simulink model "final_quadruped_140622_veldelay"  (R2021a)
settings: Solver=ode15s  StartTime=0.0  StopTime=10  FixedStep=1e-3  RelTol=1e-5  EnableMultiTasking=on
values from neighbouring files (symbols this model uses):
  foot_x = 8    [bipedparameters.m]    (also in fcn.m; finalrobotParameters.m; finalrobotParameters_110522.m; finalrobotParameters_140522.m)
  foot_y = 6    [bipedparameters.m]    (also in fcn.m; finalrobotParameters.m; finalrobotParameters_110522.m; finalrobotParameters_140522.m)
  foot_z = 1    [bipedparameters.m]    (also in fcn.m; finalrobotParameters.m; finalrobotParameters_110522.m; finalrobotParameters_140522.m)
  height_plane = 0.025    [bipedparameters.m]    (also in finalrobotParameters.m; finalrobotParameters_110522.m; finalrobotParameters_140522.m; finalrobotParameters_240522.m)
  kd_ankle = 1000    [bipedparameters.m]    (also in finalrobotParameters_240522.m)
  kd_hip = 1000    [bipedparameters.m]    (also in finalrobotParameters_240522.m)
  kd_knee = 1000    [bipedparameters.m]    (also in finalrobotParameters_240522.m)
  ki_ankle = 1000    [bipedparameters.m]    (also in finalrobotParameters_240522.m)
  ki_hip = 1000    [bipedparameters.m]    (also in finalrobotParameters_240522.m)
  ki_knee = 2000    [bipedparameters.m]    (also in finalrobotParameters_240522.m)
  kp_ankle = 1000    [bipedparameters.m]    (also in finalrobotParameters_240522.m)
  kp_hip = 1000    [bipedparameters.m]    (also in finalrobotParameters_240522.m)
  kp_knee = 2000    [bipedparameters.m]    (also in finalrobotParameters_240522.m)
  lower_leg_length = 10    [bipedparameters.m]    (also in fcn.m; finalrobotParameters.m; finalrobotParameters_110522.m; finalrobotParameters_140522.m)
  m_ll = density*leg_radius*leg_radius*lower_leg_length*3.141592653589*0.01*0.01*0.01    (= 0.0176714586764)    [bipedparameters.m]    (also in fcn.m; finalrobotParameters_140522.m; finalrobotParameters_240522.m; hdotlb.m)
  m_ul = density*leg_radius*leg_radius*upper_leg_length*3.141592653589*0.01*0.01*0.01    (= 0.0176714586764)    [bipedparameters.m]    (also in fcn.m; finalrobotParameters_140522.m; finalrobotParameters_240522.m; hdotlb.m)
  plane_x = 25    [bipedparameters.m]    (also in finalrobotParameters.m; finalrobotParameters_110522.m; finalrobotParameters_140522.m; finalrobotParameters_240522.m)
  plane_y = 3    [bipedparameters.m]    (also in finalrobotParameters.m; finalrobotParameters_110522.m; finalrobotParameters_140522.m; finalrobotParameters_240522.m)
  torso_offset_x = -0.5    [bipedparameters.m]    (also in finalrobotParameters.m = 10; finalrobotParameters_110522.m = 10; finalrobotParameters_140522.m = 10; finalrobotParameters_240522.m = 10)
  torso_offset_z = -2    [bipedparameters.m]    (also in finalrobotParameters.m; finalrobotParameters_110522.m; finalrobotParameters_140522.m; finalrobotParameters_240522.m)
  torso_x = 5    [bipedparameters.m]    (also in fcn.m = 25; finalrobotParameters.m = 25; finalrobotParameters_110522.m = 25; finalrobotParameters_140522.m = 25)
  torso_y = 10    [bipedparameters.m]    (also in fcn.m = 16; finalrobotParameters.m = 16; finalrobotParameters_110522.m = 16; finalrobotParameters_140522.m = 16)
  torso_z = 8    [bipedparameters.m]    (also in fcn.m = 10; finalrobotParameters.m = 10; finalrobotParameters_110522.m = 10; finalrobotParameters_140522.m = 10)
  upper_leg_length = 10    [bipedparameters.m]    (also in fcn.m; finalrobotParameters.m; finalrobotParameters_110522.m; finalrobotParameters_140522.m)
undefined symbols (not defined in the file or in its folder): X, Y, Z
libraries: nesl_utility x151, sm_lib x71, Contact_Forces_Lib x16, pid_lib x12, fl_lib x4
(part 7 of 7)

== matlab function final_quadruped_140622_veldelay/Model/Left Leg Front/Subsystem/MATLAB Function1 ==
  data: eb10g input; eb20g input; ab10g input; cmb2 input; cmb1 input; cmb3 input; eb30g input; hLF output; ab20g input; rhoLF output
function [hLF,rhoLF] = fcn(eb10g, eb20g, ab10g, cmb2, cmb1, cmb3, eb30g, ab20g)
%%
lower_leg_length = 10;
upper_leg_length = 10;
density = 1000;
foot_density=2000;
leg_radius = 0.75;
foot_x = 8;
foot_y = 6;
foot_z = 1;
m_ul=density*leg_radius*leg_radius*upper_leg_length*3.141592653589*0.01*0.01*0.01;
m_ll=density*leg_radius*leg_radius*lower_leg_length*3.141592653589*0.01*0.01*0.01;
m_foot=foot_density*foot_x*foot_y*foot_z*0.000001;
%%
scf=zeros(3,3);
sof=zeros(3,3);
rhoLF=zeros(3,3,3);
scf(:,1)=cmb1;
scf(:,2)=ab10g+cmb2;
scf(:,3)=ab10g+ab20g+cmb3;
sof(:,1)=[0;0;0];
sof(:,2)=ab10g;
sof(:,3)=ab10g+ab20g;
for i=1:3
    for j=1:3
        if j<i
rhoLF(:,j,i)=zeros(3,1);
        else
rhoLF(:,j,i)=scf(:,j)-sof(:,i);
        end
    end
end
h1=(m_ul*cross(eb10g,rhoLF(:,1,1)))+(m_ll*cross(eb10g,rhoLF(:,2,1)))+(m_foot*cross(eb10g,rhoLF(:,3,1)));
h2=(m_ll*cross(eb20g,rhoLF(:,2,2)))+(m_foot*cross(eb20g,rhoLF(:,3,2)));
h3=m_foot*(cross(eb30g,rhoLF(:,3,3)));

hLF =[h1 h2 h3];



end

== matlab function final_quadruped_140622_veldelay/Model/Right Leg Back/Subsystem/MATLAB Function1 ==
  data: ec10g input; ec20g input; ac10g input; cmc2 input; cmc1 input; cmc3 input; ec30g input; ac20g input; hRB output; rhoRB output
function [hRB,rhoRB] = fcn(ec10g, ec20g, ac10g, cmc2, cmc1, cmc3, ec30g, ac20g)
%%
lower_leg_length = 10;
upper_leg_length = 10;
density = 1000;
foot_density=2000;
leg_radius = 0.75;
foot_x = 8;
foot_y = 6;
foot_z = 1;
m_ul=density*leg_radius*leg_radius*upper_leg_length*3.141592653589*0.01*0.01*0.01;
m_ll=density*leg_radius*leg_radius*lower_leg_length*3.141592653589*0.01*0.01*0.01;
m_foot=foot_density*foot_x*foot_y*foot_z*0.000001;
%%
scf=zeros(3,3);
sof=zeros(3,3);
rhoRB=zeros(3,3,3);
scf(:,1)=cmc1;
scf(:,2)=ac10g+cmc2;
scf(:,3)=ac10g+ac20g+cmc3;
sof(:,1)=[0;0;0];
sof(:,2)=ac10g;
sof(:,3)=ac10g+ac20g;
for i=1:3
    for j=1:3
        if j<i
rhoRB(:,j,i)=zeros(3,1);
        else
rhoRB(:,j,i)=scf(:,j)-sof(:,i);
        end
    end
end
h1=(m_ul*cross(ec10g,rhoRB(:,1,1)))+(m_ll*cross(ec10g,rhoRB(:,2,1)))+(m_foot*cross(ec10g,rhoRB(:,3,1)));
h2=(m_ll*cross(ec20g,rhoRB(:,2,2)))+(m_foot*cross(ec20g,rhoRB(:,3,2)));
h3=m_foot*(cross(ec30g,rhoRB(:,3,3)));

hRB =[h1 h2 h3];



end

== matlab function final_quadruped_140622_veldelay/Model/Left LegBack/Subsystem/MATLAB Function1 ==
  data: ed10g input; ed20g input; ad10g input; cmd2 input; cmd1 input; cmd3 input; ed30g input; ad20g input; hLB output; rhoLB output
function [hLB,rhoLB] = fcn(ed10g, ed20g, ad10g, cmd2, cmd1, cmd3, ed30g, ad20g)
%%
lower_leg_length = 10;
upper_leg_length = 10;
density = 1000;
foot_density=2000;
leg_radius = 0.75;
foot_x = 8;
foot_y = 6;
foot_z = 1;
m_ul=density*leg_radius*leg_radius*upper_leg_length*3.141592653589*0.01*0.01*0.01;
m_ll=density*leg_radius*leg_radius*lower_leg_length*3.141592653589*0.01*0.01*0.01;
m_foot=foot_density*foot_x*foot_y*foot_z*0.000001;
%%
scf=zeros(3,3);
sof=zeros(3,3);
rhoLB=zeros(3,3,3);
scf(:,1)=cmd1;
scf(:,2)=ad10g+cmd2;
scf(:,3)=ad10g+ad20g+cmd3;
sof(:,1)=[0;0;0];
sof(:,2)=ad10g;
sof(:,3)=ad10g+ad20g;
for i=1:3
    for j=1:3
        if j<i
rhoLB(:,j,i)=zeros(3,1);
        else
rhoLB(:,j,i)=scf(:,j)-sof(:,i);
        end
    end
end
h1=(m_ul*cross(ed10g,rhoLB(:,1,1)))+(m_ll*cross(ed10g,rhoLB(:,2,1)))+(m_foot*cross(ed10g,rhoLB(:,3,1)));
h2=(m_ll*cross(ed20g,rhoLB(:,2,2)))+(m_foot*cross(ed20g,rhoLB(:,3,2)));
h3=m_foot*(cross(ed30g,rhoLB(:,3,3)));

hLB =[h1 h2 h3];



end

== matlab function final_quadruped_140622_veldelay/MATLAB Function ==
  data: vx input; v_torso output; vy input; vz input
function v_torso = fcn(vx, vy, vz)
v_torso=[vx; vy; vz];
end

== matlab function final_quadruped_140622_veldelay/Model/Right Leg Front /MATLAB Function2 ==
  data: tddRF input; tddRF_hip output; tddRF_knee output; tddRF_ankle output
function [tddRF_hip, tddRF_knee, tddRF_ankle] = fcn(tddRF)
tddRF_hip=tddRF(1);
tddRF_knee=tddRF(2);
tddRF_ankle=tddRF(3);
end

== matlab function final_quadruped_140622_veldelay/Model/Left Leg Front/MATLAB Function2 ==
  data: tddLF input; tddLF_hip output; tddLF_knee output; tddLF_ankle output
function [tddLF_hip, tddLF_knee, tddLF_ankle] = fcn(tddLF)
tddLF_hip=tddLF(1);
tddLF_knee=tddLF(2);
tddLF_ankle=tddLF(3);
end

== matlab function final_quadruped_140622_veldelay/Model/Right Leg Back/MATLAB Function2 ==
  data: tddRB input; tddRB_hip output; tddRB_knee output; tddRB_ankle output
function [tddRB_hip, tddRB_knee, tddRB_ankle] = fcn(tddRB)
tddRB_hip=tddRB(1);
tddRB_knee=tddRB(2);
tddRB_ankle=tddRB(3);
end

== matlab function final_quadruped_140622_veldelay/Model/Left LegBack/MATLAB Function2 ==
  data: tddLB input; tddLB_hip output; tddLB_knee output; tddLB_ankle output
function [tddLB_hip, tddLB_knee, tddLB_ankle] = fcn(tddLB)
tddLB_hip=tddLB(1);
tddLB_knee=tddLB(2);
tddLB_ankle=tddLB(3);
end

== matlab function final_quadruped_140622_veldelay/Subsystem/MATLAB Function4 ==
  data: vx input; vy input; v output; vz input; ax input; ay input; az input; a output
function [v,a] = fcn(vx,vy,vz,ax,ay,az)
v=[vx;vy;vz];
a=[ax;ay;az];
end

== matlab function final_quadruped_140622_veldelay/Subsystem/MATLAB Function1 ==
  data: vx input; vy input; v output; vz input; ax input; ay input; az input; a output
function [v,a] = fcn(vx,vy,vz,ax,ay,az)
v=[vx;vy;vz];
a=[ax;ay;az];
end

== matlab function final_quadruped_140622_veldelay/Subsystem/MATLAB Function5 ==
  data: vx input; vy input; v output; vz input; ax input; ay input; az input; a output
function [v,a] = fcn(vx,vy,vz,ax,ay,az)
v=[vx;vy;vz];
a=[ax;ay;az];
end

== matlab function final_quadruped_140622_veldelay/Subsystem/MATLAB Function6 ==
  data: vx input; vy input; v output; vz input; ax input; ay input; az input; a output
function [v,a] = fcn(vx,vy,vz,ax,ay,az)
v=[vx;vy;vz];
a=[ax;ay;az];
end

== matlab function final_quadruped_140622_veldelay/Subsystem/MATLAB Function7 ==
  data: vx input; vy input; v output; vz input; ax input; ay input; az input; a output
function [v,a] = fcn(vx,vy,vz,ax,ay,az)
v=[vx;vy;vz];
a=[ax;ay;az];
end

== matlab function final_quadruped_140622_veldelay/Subsystem/MATLAB Function8 ==
  data: vx input; vy input; v output; vz input; ax input; ay input; az input; a output
function [v,a] = fcn(vx,vy,vz,ax,ay,az)
v=[vx;vy;vz];
a=[ax;ay;az];
end

== matlab function final_quadruped_140622_veldelay/Subsystem/MATLAB Function9 ==
  data: vx input; vy input; v output; vz input; ax input; ay input; az input; a output
function [v,a] = fcn(vx,vy,vz,ax,ay,az)
v=[vx;vy;vz];
a=[ax;ay;az];
end

== matlab function final_quadruped_140622_veldelay/Subsystem/MATLAB Function10 ==
  data: vx input; vy input; v output; vz input; ax input; ay input; az input; a output
function [v,a] = fcn(vx,vy,vz,ax,ay,az)
v=[vx;vy;vz];
a=[ax;ay;az];
end

== matlab function final_quadruped_140622_veldelay/Subsystem/MATLAB Function11 ==
  data: vx input; vy input; v output; vz input; ax input; ay input; az input; a output
function [v,a] = fcn(vx,vy,vz,ax,ay,az)
v=[vx;vy;vz];
a=[ax;ay;az];
end

== matlab function final_quadruped_140622_veldelay/Subsystem/MATLAB Function12 ==
  data: vx input; vy input; v output; vz input; ax input; ay input; az input; a output
function [v,a] = fcn(vx,vy,vz,ax,ay,az)
v=[vx;vy;vz];
a=[ax;ay;az];
end

== matlab function final_quadruped_140622_veldelay/Subsystem/MATLAB Function14 ==
  data: vx input; vy input; v output; vz input; ax input; ay input; az input; a output
function [v,a] = fcn(vx,vy,vz,ax,ay,az)
v=[vx;vy;vz];
a=[ax;ay;az];
end

== matlab function final_quadruped_140622_veldelay/Model/Right Leg Front /MATLAB Function ==
  data: ankle input; knee input; tdRF output; hip input
function tdRF= fcn(ankle, knee, hip)
tdRF=[hip;knee;ankle];
end

== matlab function final_quadruped_140622_veldelay/Subsystem/MATLAB Function13 ==
  data: vulRF input; vllRF input; Mvcm output; vfRF input; vulLF input; vllLF input; vfLF input; vulRB input; vllRB input; vfRB input; vulLB input; vllLB input; vfLB input; v_torso input; vlinks output; vcm output
function [Mvcm,vlinks,vcm] = fcn(vulRF,vllRF,vfRF,vulLF,vllLF,vfLF,vulRB,vllRB,vfRB,vulLB,vllLB,vfLB,v_torso)
%%
lower_leg_length = 10;
upper_leg_length = 10;
density = 1000;
foot_density=2000;
leg_radius = 0.75;
foot_x = 8;
foot_y = 6;
foot_z = 1;
torso_y = 16;
torso_x = 25;
torso_z = 10;
m_ul=density*leg_radius*leg_radius*upper_leg_length*3.141592653589*0.01*0.01*0.01;
m_ll=density*leg_radius*leg_radius*lower_leg_length*3.141592653589*0.01*0.01*0.01;
m_foot=foot_density*foot_x*foot_y*foot_z*0.000001;
m_torso=density*torso_x*torso_y*torso_z*0.000001;
M=m_torso+4*(m_ul+m_ll+m_foot);
%%
Mvcm=m_torso*v_torso+(m_ul*vulRF+m_ll*vllRF+m_foot*vfRF)+(m_ul*vulLF+m_ll*vllLF+m_foot*vfLF)+(m_ul*vulRB+m_ll*vllRB+m_foot*vfRB)+(m_ul*vulLB+m_ll*vllLB+m_foot*vfLB);
vlinks=[vulRF vllRF vfRF vulLF vllLF vfLF vulRB vllRB vfRB vulLB vllLB vfLB];
vcm=Mvcm/M;
end

== matlab function final_quadruped_140622_veldelay/Model/Left Leg Front/MATLAB Function ==
  data: ankle input; knee input; tdRF output; hip input
function tdRF= fcn(ankle, knee, hip)
tdRF=[hip;knee;ankle];
end

== matlab function final_quadruped_140622_veldelay/Model/Right Leg Back/MATLAB Function ==
  data: ankle input; knee input; tdRF output; hip input
function tdRF= fcn(ankle, knee, hip)
tdRF=[hip;knee;ankle];
end

== matlab function final_quadruped_140622_veldelay/Model/Left LegBack/MATLAB Function ==
  data: ankle input; knee input; tdLB output; hip input
function tdLB= fcn(ankle, knee, hip)
tdLB=[hip;knee;ankle];
end

== matlab function final_quadruped_140622_veldelay/Model/MATLAB Function ==
  data: tdRF input; td output; tdLF input; tdRB input; tdLB input; t2dRF input; t2dLF input; t2dRB input; t2dLB input; t2d output
function [td,t2d] = fcn(tdRF,tdLF,tdRB,tdLB,t2dRF,t2dLF,t2dRB,t2dLB)
td=[tdRF;tdLF;tdRB;tdLB];
t2d=[t2dRF;t2dLF;t2dRB;t2dLB];
end

== matlab function final_quadruped_140622_veldelay/Model/MATLAB Function1 ==
  data: h input; h_dot input; ht2d output; td input; t2d input; h_dottd output; htd output; theta_d_des input; theta_2d_des input; ht2ddes output; hdtddes output
function [ht2d,h_dottd,htd,ht2ddes,hdtddes] = fcn(h,h_dot, td, t2d,theta_d_des,theta_2d_des)
ht2d=h*t2d;
htd=h*td;
h_dottd=h_dot*td;
ht2ddes=h*theta_2d_des;
hdtddes=h_dot*theta_d_des;
end

== matlab function final_quadruped_140622_veldelay/MATLAB Function1 ==
  data: Mvcm input; error output; ht2d input; h_dottd input; a_torso input; v_torso input; f input; Macm input; htd input; ht2ddes input; hdtddes input; v_error output; theta_d_des input; h input; v_error_eig output
function [error, v_error,v_error_eig] = fcn(Mvcm,ht2d,h_dottd,a_torso, v_torso, f,Macm,htd, ht2ddes, hdtddes, theta_d_des,h)
%%
lower_leg_length = 10;
upper_leg_length = 10;
density = 1000;
foot_density=2000;
leg_radius = 0.75;
foot_x = 8;
foot_y = 6;
foot_z = 1;
torso_y = 16;
torso_x = 25;
torso_z = 10;
m_ul=density*leg_radius*leg_radius*upper_leg_length*3.141592653589*0.01*0.01*0.01;
m_ll=density*leg_radius*leg_radius*lower_leg_length*3.141592653589*0.01*0.01*0.01;
m_foot=foot_density*foot_x*foot_y*foot_z*0.000001;
m_torso=density*torso_x*torso_y*torso_z*0.000001;
M=m_torso+(4*(m_ul+m_ll+m_foot));
g=[0; 0; -9.80067];
%%
%v_error=htd+M*v_torso-Mvcm;
v_error=h*theta_d_des+M*v_torso-Mvcm;
v_error_eig=h*theta_d_des+M*v_torso-Mvcm;
error2=ht2d+h_dottd+M*a_torso-M*g-f-Macm;
error=ht2ddes+hdtddes+M*a_torso-M*g-f-Macm;
end

== matlab function final_quadruped_140622_veldelay/Model/Right Leg Front /Subsystem/MATLAB Function2 ==
  data: h_dotRF output; ea_dg1 input; ea1g input; ea2g input; ea3g input; ea_dg2 input; ea_dg3 input; rho_dotRF input; rhoRF input
function h_dotRF = fcn(  ea_dg1,ea1g, ea2g, ea3g, ea_dg2, ea_dg3, rho_dotRF, rhoRF)
%%
lower_leg_length = 10;
upper_leg_length = 10;
density = 1000;
foot_density=2000;
leg_radius = 0.75;
foot_x = 8;
foot_y = 6;
foot_z = 1;
m_ul=density*leg_radius*leg_radius*upper_leg_length*3.141592653589*0.01*0.01*0.01;
m_ll=density*leg_radius*leg_radius*lower_leg_length*3.141592653589*0.01*0.01*0.01;
m_foot=foot_density*foot_x*foot_y*foot_z*0.000001;

%%
h1_dot=(m_ul*cross(ea1g,rho_dotRF(:,1,1)))+(m_ul*cross(ea_dg1,rhoRF(:,1,1)))+(m_ll*cross(ea1g,rho_dotRF(:,2,1)))+(m_ll*cross(ea_dg1,rhoRF(:,2,1)))+(m_foot*cross(ea1g,rho_dotRF(:,3,1)))+(m_foot*cross(ea_dg1,rhoRF(:,3,1)));
h2_dot=(m_ll*cross(ea2g,rho_dotRF(:,2,2)))+(m_ll*cross(ea_dg2,rhoRF(:,2,2)))+(m_foot*cross(ea2g,rho_dotRF(:,3,2)))+(m_foot*cross(ea_dg2,rhoRF(:,3,2)));
h3_dot=m_foot*(cross(ea3g,rho_dotRF(:,3,3)))+m_foot*(cross(ea_dg3,rhoRF(:,3,3)));

h_dotRF =[h1_dot h2_dot h3_dot];



end

== matlab function final_quadruped_140622_veldelay/Model/Left Leg Front/Subsystem/MATLAB Function2 ==
  data: h_dotLF output; eb_dg1 input; eb1g input; eb2g input; eb3g input; eb_dg2 input; eb_dg3 input; rho_dotLF input; rhoLF input
function h_dotLF = fcn( eb_dg1,eb1g, eb2g, eb3g, eb_dg2, eb_dg3, rho_dotLF, rhoLF)
%%
lower_leg_length = 10;
upper_leg_length = 10;
density = 1000;
foot_density=2000;
leg_radius = 0.75;
foot_x = 8;
foot_y = 6;
foot_z = 1;
m_ul=density*leg_radius*leg_radius*upper_leg_length*3.141592653589*0.01*0.01*0.01;
m_ll=density*leg_radius*leg_radius*lower_leg_length*3.141592653589*0.01*0.01*0.01;
m_foot=foot_density*foot_x*foot_y*foot_z*0.000001;

%%
h1_dot=(m_ul*cross(eb1g,rho_dotLF(:,1,1)))+(m_ul*cross(eb_dg1,rhoLF(:,1,1)))+(m_ll*cross(eb1g,rho_dotLF(:,2,1)))+(m_ll*cross(eb_dg1,rhoLF(:,2,1)))+(m_foot*cross(eb1g,rho_dotLF(:,3,1)))+(m_foot*cross(eb_dg1,rhoLF(:,3,1)));
h2_dot=(m_ll*cross(eb2g,rho_dotLF(:,2,2)))+(m_ll*cross(eb_dg2,rhoLF(:,2,2)))+(m_foot*cross(eb2g,rho_dotLF(:,3,2)))+(m_foot*cross(eb_dg2,rhoLF(:,3,2)));
h3_dot=m_foot*(cross(eb3g,rho_dotLF(:,3,3)))+m_foot*(cross(eb_dg3,rhoLF(:,3,3)));

h_dotLF =[h1_dot h2_dot h3_dot];



end

== matlab function final_quadruped_140622_veldelay/Model/Right Leg Front /Subsystem/MATLAB Function4 ==
  data: ea1g input; ea2g input; aa1g input; aa2g input; ea3g input; vlinks input; w_torso input; ea_dg1 output; td1 input; v_torso input; ea_dg2 output; td2 input; td3 input; ea_dg3 output; rho_dotRF output
function [ea_dg1,ea_dg2,ea_dg3,rho_dotRF] = fcn(ea1g,ea2g,aa1g,aa2g, ea3g, vlinks, w_torso, td1, v_torso, td2, td3)
w0=w_torso;
w1=w0+ea1g*td1;
w2=w1+ea2g*td2;
w3=w2+ea3g*td3;
%e dot = omega X e
ea_dg1=cross(w1,ea1g);
ea_dg2=cross(w2,ea2g);
ea_dg3=cross(w3,ea3g);


vcf=zeros(3,3);
vof=zeros(3,3);
rho_dotRF=zeros(3,3,3);
vcf(:,1)=vlinks(1);
vcf(:,2)=vlinks(2);
vcf(:,3)=vlinks(3);
vof(:,1)=v_torso;
vof(:,2)=vof(:,1)+cross(w1,aa1g);
vof(:,3)=vof(:,2)+cross(w2,aa2g);
for i=1:3
    for j=1:3
        if j<i
rho_dotRF(:,j,i)=zeros(3,1);
        else
rho_dotRF(:,j,i)=vcf(:,j)-vof(:,i);
        end
    end
end

end

== matlab function final_quadruped_140622_veldelay/Model/Left Leg Front/Subsystem/MATLAB Function4 ==
  data: eb1g input; eb2g input; ab1g input; ab2g input; eb3g input; vlinks input; w_torso input; eb_dg1 output; td1 input; v_torso input; eb_dg2 output; td2 input; td3 input; eb_dg3 output; rho_dotLF output
function [eb_dg1,eb_dg2,eb_dg3,rho_dotLF] = fcn(eb1g,eb2g,ab1g,ab2g, eb3g, vlinks, w_torso, td1, v_torso, td2, td3)
w0=w_torso;
w1=w0+eb1g*td1;
w2=w1+eb2g*td2;
w3=w2+eb3g*td3;

eb_dg1=cross(w1,eb1g);
eb_dg2=cross(w2,eb2g);
eb_dg3=cross(w3,eb3g);


vcf=zeros(3,3);
vof=zeros(3,3);
rho_dotLF=zeros(3,3,3);
vcf(:,1)=vlinks(4);
vcf(:,2)=vlinks(5);
vcf(:,3)=vlinks(6);
vof(:,1)=v_torso;
vof(:,2)=vof(:,1)+cross(w1,ab1g);
vof(:,3)=vof(:,2)+cross(w2,ab2g);
for i=1:3
    for j=1:3
        if j<i
rho_dotLF(:,j,i)=zeros(3,1);
        else
rho_dotLF(:,j,i)=vcf(:,j)-vof(:,i);
        end
    end
end

end

== matlab function final_quadruped_140622_veldelay/Model/Right Leg Back/Subsystem/MATLAB Function2 ==
  data: h_dotRB output; ec_dg1 input; ec1g input; ec2g input; ec3g input; ec_dg2 input; ec_dg3 input; rho_dotRB input; rhoRB input
function h_dotRB = fcn( ec_dg1,ec1g, ec2g, ec3g, ec_dg2, ec_dg3, rho_dotRB, rhoRB)
%%
lower_leg_length = 10;
upper_leg_length = 10;
density = 1000;
foot_density=2000;
leg_radius = 0.75;
foot_x = 8;
foot_y = 6;
foot_z = 1;
m_ul=density*leg_radius*leg_radius*upper_leg_length*3.141592653589*0.01*0.01*0.01;
m_ll=density*leg_radius*leg_radius*lower_leg_length*3.141592653589*0.01*0.01*0.01;
m_foot=foot_density*foot_x*foot_y*foot_z*0.000001;

%%
h1_dot=(m_ul*cross(ec1g,rho_dotRB(:,1,1)))+(m_ul*cross(ec_dg1,rhoRB(:,1,1)))+(m_ll*cross(ec1g,rho_dotRB(:,2,1)))+(m_ll*cross(ec_dg1,rhoRB(:,2,1)))+(m_foot*cross(ec1g,rho_dotRB(:,3,1)))+(m_foot*cross(ec_dg1,rhoRB(:,3,1)));
h2_dot=(m_ll*cross(ec2g,rho_dotRB(:,2,2)))+(m_ll*cross(ec_dg2,rhoRB(:,2,2)))+(m_foot*cross(ec2g,rho_dotRB(:,3,2)))+(m_foot*cross(ec_dg2,rhoRB(:,3,2)));
h3_dot=m_foot*(cross(ec3g,rho_dotRB(:,3,3)))+m_foot*(cross(ec_dg3,rhoRB(:,3,3)));

h_dotRB =[h1_dot h2_dot h3_dot];



end

== matlab function final_quadruped_140622_veldelay/Model/Right Leg Back/Subsystem/MATLAB Function4 ==
  data: ec1g input; ec2g input; ac1g input; ac2g input; ec3g input; vlinks input; w_torso input; ec_dg1 output; td1 input; v_torso input; ec_dg2 output; td2 input; td3 input; ec_dg3 output; rho_dotRB output
function [ec_dg1,ec_dg2,ec_dg3,rho_dotRB] = fcn(ec1g,ec2g,ac1g,ac2g, ec3g, vlinks, w_torso, td1, v_torso, td2, td3)
w0=w_torso;
w1=w0+ec1g*td1;
w2=w1+ec2g*td2;
w3=w2+ec3g*td3;

ec_dg1=cross(w1,ec1g);
ec_dg2=cross(w2,ec2g);
ec_dg3=cross(w3,ec3g);


vcf=zeros(3,3);
vof=zeros(3,3);
rho_dotRB=zeros(3,3,3);
vcf(:,1)=vlinks(7);
vcf(:,2)=vlinks(8);
vcf(:,3)=vlinks(9);
vof(:,1)=v_torso;
vof(:,2)=vof(:,1)+cross(w1,ac1g);
vof(:,3)=vof(:,2)+cross(w2,ac2g);
for i=1:3
    for j=1:3
        if j<i
rho_dotRB(:,j,i)=zeros(3,1);
        else
rho_dotRB(:,j,i)=vcf(:,j)-vof(:,i);
        end
    end
end

end

== matlab function final_quadruped_140622_veldelay/Model/Left LegBack/Subsystem/MATLAB Function2 ==
  data: h_dotLB output; ed_dg1 input; ed1g input; ed2g input; ed3g input; ed_dg2 input; ed_dg3 input; rho_dotLB input; rhoLB input
function h_dotLB = fcn( ed_dg1,ed1g, ed2g, ed3g, ed_dg2, ed_dg3, rho_dotLB, rhoLB)
%%
lower_leg_length = 10;
upper_leg_length = 10;
density = 1000;
foot_density=2000;
leg_radius = 0.75;
foot_x = 8;
foot_y = 6;
foot_z = 1;
m_ul=density*leg_radius*leg_radius*upper_leg_length*3.141592653589*0.01*0.01*0.01;
m_ll=density*leg_radius*leg_radius*lower_leg_length*3.141592653589*0.01*0.01*0.01;
m_foot=foot_density*foot_x*foot_y*foot_z*0.000001;

%%
h1_dot=(m_ul*cross(ed1g,rho_dotLB(:,1,1)))+(m_ul*cross(ed_dg1,rhoLB(:,1,1)))+(m_ll*cross(ed1g,rho_dotLB(:,2,1)))+(m_ll*cross(ed_dg1,rhoLB(:,2,1)))+(m_foot*cross(ed1g,rho_dotLB(:,3,1)))+(m_foot*cross(ed_dg1,rhoLB(:,3,1)));
h2_dot=(m_ll*cross(ed2g,rho_dotLB(:,2,2)))+(m_ll*cross(ed_dg2,rhoLB(:,2,2)))+(m_foot*cross(ed2g,rho_dotLB(:,3,2)))+(m_foot*cross(ed_dg2,rhoLB(:,3,2)));
h3_dot=m_foot*(cross(ed3g,rho_dotLB(:,3,3)))+m_foot*(cross(ed_dg3,rhoLB(:,3,3)));

h_dotLB =[h1_dot h2_dot h3_dot];



end

== matlab function final_quadruped_140622_veldelay/Model/Left LegBack/Subsystem/MATLAB Function4 ==
  data: ed1g input; ed2g input; ad1g input; ad2g input; ed3g input; vlinks input; w_torso input; ed_dg1 output; td1 input; v_torso input; ed_dg2 output; td2 input; td3 input; ed_dg3 output; rho_dotLB output
function [ed_dg1,ed_dg2,ed_dg3,rho_dotLB] = fcn(ed1g,ed2g,ad1g,ad2g, ed3g, vlinks, w_torso, td1, v_torso, td2, td3)
w0=w_torso;
w1=w0+ed1g*td1;
w2=w1+ed2g*td2;
w3=w2+ed3g*td3;

ed_dg1=cross(w1,ed1g);
ed_dg2=cross(w2,ed2g);
ed_dg3=cross(w3,ed3g);


vcf=zeros(3,3);
vof=zeros(3,3);
rho_dotLB=zeros(3,3,3);
vcf(:,1)=vlinks(10);
vcf(:,2)=vlinks(11);
vcf(:,3)=vlinks(12);
vof(:,1)=v_torso;
vof(:,2)=vof(:,1)+cross(w1,ad1g);
vof(:,3)=vof(:,2)+cross(w2,ad2g);
for i=1:3
    for j=1:3
        if j<i
rho_dotLB(:,j,i)=zeros(3,1);
        else
rho_dotLB(:,j,i)=vcf(:,j)-vof(:,i);
        end
    end
end

end

== matlab function final_quadruped_140622_veldelay/Subsystem/MATLAB Function2 ==
  data: vx input; vy input; v output; vz input; ax input; ay input; az input; a output
function [v,a] = fcn(vx,vy,vz,ax,ay,az)
v=[vx;vy;vz];
a=[ax;ay;az];
end

== matlab function final_quadruped_140622_veldelay/Model/Left Leg Front/MATLAB Function1 ==
  data: ankle input; knee input; t2dLF output; hip input
function t2dLF= fcn(ankle, knee, hip)
t2dLF=[hip;knee;ankle];
end

== matlab function final_quadruped_140622_veldelay/Model/Right Leg Front /MATLAB Function1 ==
  data: ankle input; knee input; t2dRF output; hip input
function t2dRF= fcn(ankle, knee, hip)
t2dRF=[hip;knee;ankle];
end

== matlab function final_quadruped_140622_veldelay/MATLAB Function2 ==
  data: ax input; a_torso output; ay input; az input
function a_torso = fcn(ax, ay, az)
a_torso=[ax(1); ay(1); az(1)];
end

== matlab function final_quadruped_140622_veldelay/Model/Left Leg Front/Contact Forces /MATLAB Function ==
  data: n1 input; NLF output; n2 input; n4 input; n3 input; f1 input; f2 input; f3 input; f4 input; FLF output; Qd3g input
function [NLF,FLF] = fcn(n1,n2,n4,n3,f1,f2,f3,f4, Qd3g)
Qds3=[1 0 0;
      0 cos(90) -sin(90);
      0 sin(90) cos(90)];
% mu_s = 0.8;
% alpha=atan(mu_s);
% NRF=n1+n2+n3+n4;
% FRFca=f1*cos(alpha)+f2*cos(alpha)+f3*cos(alpha)+f4*cos(alpha);
% FRFsa=f1*sin(alpha)+f2*sin(alpha)+f3*sin(alpha)+f4*sin(alpha);
NLF=n1+n2+n3+n4;
FLF=f1+f2+f3+f4;
FLF=Qds3*Qd3g*FLF;
end

== matlab function final_quadruped_140622_veldelay/Model/MATLAB Function2 ==
  data: theta_d_des input; theta_2d_des output; h_dot input; h input; a_torso input; M input; f input
function theta_2d_des = fcn(theta_d_des, h_dot, h, a_torso, M, f)
g=[0; 0; -9.80665];
theta_2d_des=pinv(h)*((-h_dot*theta_d_des)-M*a_torso+M*g+f);
end

== matlab function final_quadruped_140622_veldelay/Model/Right Leg Front /Contact Forces /MATLAB Function ==
  data: n1 input; NRF output; n2 input; n4 input; n3 input; f1 input; f2 input; f3 input; f4 input; FRF output; Qd3g input
function [NRF,FRF] = fcn(n1,n2,n4,n3,f1,f2,f3,f4, Qd3g)
% mu_s = 0.8;
% alpha=atan(mu_s);
% NRF=n1+n2+n3+n4;
% FRFca=f1*cos(alpha)+f2*cos(alpha)+f3*cos(alpha)+f4*cos(alpha);
% FRFsa=f1*sin(alpha)+f2*sin(alpha)+f3*sin(alpha)+f4*sin(alpha);
Qds3=[1 0 0;
      0 cos(90) -sin(90);
      0 sin(90) cos(90)];
NRF=n1+n2+n3+n4;
FRFl=f1+f2+f3+f4;
FRF=Qds3*Qd3g*FRFl;
end

== matlab function final_quadruped_140622_veldelay/Model/Right Leg Back/Contact Forces /MATLAB Function ==
  data: n1 input; NRB output; n2 input; n4 input; n3 input; f1 input; f2 input; f3 input; f4 input; FRB output; Qd3g input
function [NRB,FRB] = fcn(n1,n2,n4,n3,f1,f2,f3,f4,Qd3g)
Qds3=[1 0 0;
      0 cos(90) -sin(90);
      0 sin(90) cos(90)];
% mu_s = 0.8;
% alpha=atan(mu_s);
% NRF=n1+n2+n3+n4;
% FRFca=f1*cos(alpha)+f2*cos(alpha)+f3*cos(alpha)+f4*cos(alpha);
% FRFsa=f1*sin(alpha)+f2*sin(alpha)+f3*sin(alpha)+f4*sin(alpha);
NRB=n1+n2+n3+n4;
FRB=f1+f2+f3+f4;
FRB=Qds3*Qd3g*FRB;
end

== matlab function final_quadruped_140622_veldelay/Model/Left LegBack/Contact Forces /MATLAB Function ==
  data: n1 input; NLB output; n2 input; n4 input; n3 input; f1 input; f2 input; f3 input; f4 input; FLB output; Qd3g input
function [NLB,FLB] = fcn(n1,n2,n4,n3,f1,f2,f3,f4, Qd3g)
Qds3=[1 0 0;
      0 cos(90) -sin(90);
      0 sin(90) cos(90)];
% mu_s = 0.8;
% alpha=atan(mu_s);
% NRF=n1+n2+n3+n4;
% FRFca=f1*cos(alpha)+f2*cos(alpha)+f3*cos(alpha)+f4*cos(alpha);
% FRFsa=f1*sin(alpha)+f2*sin(alpha)+f3*sin(alpha)+f4*sin(alpha);
NLB=n1+n2+n3+n4;
FLB=f1+f2+f3+f4;
FLB=Qds3*Qd3g*FLB;
end

== matlab function final_quadruped_140622_veldelay/Model/MATLAB Function3 ==
  data: NRF input; f output; FRF input; NLF input; FLF input; NRB input; FRB input; NLB input; FLB input; N output
function [f,N] = fcn(NRF,FRF,NLF,FLF,NRB,FRB, NLB,FLB)
N=NRF+NLF+NRB+NLB;
F=FRF+FLF+FRB+FLB;
f=[-F(1);-F(2); N+F(3)];
end

== matlab function final_quadruped_140622_veldelay/Model/Right Leg Front /MATLAB Function3 ==
  data: theta_2d_des input; t2ddhip output; t2ddknee output; t2ddankle output
function [t2ddhip,t2ddknee,t2ddankle] = fcn(theta_2d_des)
t2ddhip=theta_2d_des(1);
t2ddknee=theta_2d_des(2);
t2ddankle=theta_2d_des(3);

end

== matlab function final_quadruped_140622_veldelay/Subsystem/MATLAB Function3 ==
  data: vx input; vy input; v output; vz input; ax input; ay input; az input; a output
function [v,a] = fcn(vx,vy,vz,ax,ay,az)
v=[vx;vy;vz];
a=[ax;ay;az];
end

== matlab function final_quadruped_140622_veldelay/Model/Left Leg Front/MATLAB Function3 ==
  data: theta_2d_des input; t2ddhip output; t2ddknee output; t2ddankle output
function [t2ddhip,t2ddknee,t2ddankle] = fcn(theta_2d_des)
t2ddhip=theta_2d_des(4);
t2ddknee=theta_2d_des(5);
t2ddankle=theta_2d_des(6);

end

== matlab function final_quadruped_140622_veldelay/Model/Right Leg Back/MATLAB Function3 ==
  data: theta_2d_des input; t2ddhip output; t2ddknee output; t2ddankle output
function [t2ddhip,t2ddknee,t2ddankle] = fcn(theta_2d_des)
t2ddhip=theta_2d_des(7);
t2ddknee=theta_2d_des(8);
t2ddankle=theta_2d_des(9);

end

== matlab function final_quadruped_140622_veldelay/Model/Left LegBack/MATLAB Function3 ==
  data: theta_2d_des input; t2ddhip output; t2ddknee output; t2ddankle output
function [t2ddhip,t2ddknee,t2ddankle] = fcn(theta_2d_des)
t2ddhip=theta_2d_des(10);
t2ddknee=theta_2d_des(11);
t2ddankle=theta_2d_des(12);

end

== matlab function final_quadruped_140622_veldelay/Model/Right Leg Back/MATLAB Function1 ==
  data: ankle input; knee input; t2dRF output; hip input
function t2dRF= fcn(ankle, knee, hip)
t2dRF=[hip;knee;ankle];
end

== matlab function final_quadruped_140622_veldelay/Model/Left LegBack/MATLAB Function1 ==
  data: ankle input; knee input; t2dLB output; hip input
function t2dLB= fcn(ankle, knee, hip)
t2dLB=[hip;knee;ankle];
end

== matlab function final_quadruped_140622_veldelay/Subsystem/MATLAB Function ==
  data: aulRF input; Macm output; allRF input; afRF input; aulLF input; allLF input; afLF input; aulRB input; allRB input; afRB input; aulLB input; allLB input; afLB input; a_torso input; alinks output; acm output
function [Macm,alinks,acm] = fcn(aulRF,allRF,afRF,aulLF,allLF,afLF,aulRB,allRB,afRB,aulLB,allLB,afLB,a_torso)
%%
lower_leg_length = 10;
upper_leg_length = 10;
density = 1000;
foot_density=2000;
leg_radius = 0.75;
foot_x = 8;
foot_y = 6;
foot_z = 1;
torso_y = 16;
torso_x = 25;
torso_z = 10;
m_ul=density*leg_radius*leg_radius*upper_leg_length*3.141592653589*0.01*0.01*0.01;
m_ll=density*leg_radius*leg_radius*lower_leg_length*3.141592653589*0.01*0.01*0.01;
m_foot=foot_density*foot_x*foot_y*foot_z*0.000001;
m_torso=density*torso_x*torso_y*torso_z*0.000001;
M=m_torso+4*(m_ul+m_ll+m_foot);
%%
Macm=m_torso*a_torso+(m_ul*aulRF+m_ll*allRF+m_foot*afRF)+(m_ul*aulLF+m_ll*allLF+m_foot*afLF)+(m_ul*aulRB+m_ll*allRB+m_foot*afRB)+(m_ul*aulLB+m_ll*allLB+m_foot*afLB);
alinks=[aulRF allRF afRF aulLF allLF afLF aulRB allRB afRB aulLB allLB afLB];
acm=Macm/M;
end

== matlab function final_quadruped_140622_veldelay/Model/Right Leg Front /Subsystem/MATLAB Function ==
  data: ea1g output; ea2g output; ea3g output; qha input; qaa input; Qquat input; qka input; aa1g output; aa2g output; cma1g output; cma2g output; cma3g output; Qd3g output
function [ea1g,ea2g,ea3g,aa1g,aa2g,cma1g,cma2g,cma3g,Qd3g] = fcn(qha,qaa,Qquat,qka)
%%
lower_leg_length = 10;
upper_leg_length = 10;
foot_offset=[-1; 0; 0];

%%
Qd0g=quat2rotm([Qquat(1) Qquat(2) Qquat(3) Qquat(4)]);
Qd10=[cos(qha) 0 sin(qha);
      0 1 0 ;
      -sin(qha) 0 cos(qha)];
Qd1g=Qd10*Qd0g;
  
Qd21=[cos(qka) 0 sin(qka);
      0 1 0 ;
      -sin(qka) 0 cos(qka)];
  
Qd32=[1 0 0;
      0 cos(qaa) -sin(qaa);
      0 sin(qaa) cos(qaa)];
  
Qd20 = Qd21* Qd10;
Qd30=Qd32*Qd20;
Qd2g=Qd20*Qd0g;
Qd3g=Qd30*Qd0g;

%axis in local frames
ed1l=[0;
      1;
      0];
ed2l=[0;
      1;
      0];
ed3l=[0;
     0;
     1];
  
%link vector in local frame
ad1l=[0;
      0;
      -upper_leg_length];
   
ad2l=[0;
      0;
      -lower_leg_length];
         
%axis in global frames
ea1g = Qd1g*ed1l;
ea2g = Qd2g*ed2l;
ea3g = Qd3g*ed3l;

%link vector in global frame
aa1g = Qd1g*ad1l;
aa2g = Qd2g*ad2l;

%COM distances in base frame
cma1g=aa1g/2;
cma2g=aa2g/2;
cma3g=Qd3g*foot_offset;


end
